simulink model "generate_cartesian_velocity_motion"  (R2025a)
settings: Solver=FixedStepDiscrete  StartTime=0.0  StopTime=inf  FixedStep=0.001  RelTol=1e-3
PreLoadFcn:
  | frs = FrankaRobotSettings();
libraries: simulink x1, franka_simulink x1
settings Model: SimulationMode=external  ExtModeTrigDuration=10000  Creator=vasi_ko  LastModifiedBy=kvasios
settings SolverCC: ConcurrentTasks=on  AlgebraicLoopSolver=TrustRegion
settings DataIOCC: LimitDataPoints=on  SaveFormat=Array  ReturnWorkspaceOutputs=off
settings OptimizationCC: EnhancedBackFolding=on  PassReuseOutputArgsThreshold=0.0  OptimizeBlockOrder=speed  DifferentSizesBufferReuse=on  OptimizationCustomize=off
settings DebuggingCC: SolverPrmCheckMsg=warning  ParameterTunabilityLossMsg=error  UnconnectedInputMsg=warning  UnconnectedOutputMsg=warning  UnconnectedLineMsg=warning  SFUnexpectedBacktrackingDiag=warning  SFNoUnconditionalDefaultTransitionDiag=warning  SFExecutionAtInitializationDiag=none  ArithmeticOperatorsInVariantConditions=warning
settings HardwareCC: ProdBitPerLong=64.0  ProdHWDeviceType=Intel->x86-64 (Linux 64)
settings ModelReferenceCC: EnableRefExpFcnMdlSchedulingChecks=on  PropagateSignalLabelsOutOfModel=off
settings SFSimCC: SimUseLocalCustomCode=off  MATLABDynamicMemAlloc=off  CustomCodeUndefinedFunction=UseInterfaceOnly  SimTargetLang=C++  SimDLTargetLibrary=mkl-dnn
settings RTWCC: HardwareBoard=Generic Linux AMD64 Board  RTWVerbose=off  RTWUseLocalCustomCode=off  BuildConfiguration=Faster Runs  TargetLang=C++  GPUComputeCapability=3.5  DLArmComputeVersion=19.05
settings CodeAppCC: ForceParamTrailComments=on  OperatorAnnotations=on
settings GRTTargetCC: ExtMode=on  ExtModeStaticAlloc=on  ExtModeMexFile=ext_xcp  ExtModeIntrfLevel=Level2 - Open  TargetLangStandard=C++14 (ISO)
settings ConfigComp: CovMetricSettings=dw  CovSaveCumulativeToWorkspaceVar=on  CovSaveSingleToWorkspaceVar=on  CovExternalEMLEnable=off  CovSFcnEnable=off

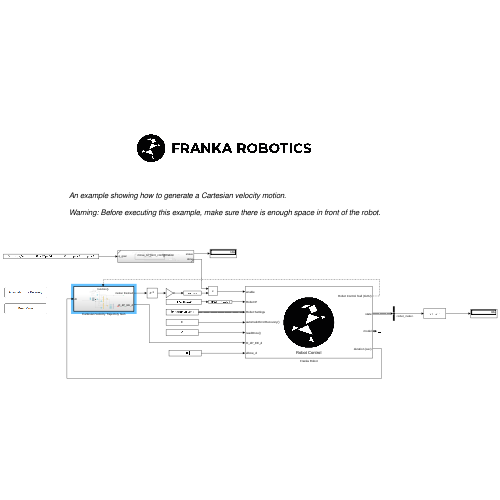
[thumbnail: Simulink's stored preview of the top-level diagram]
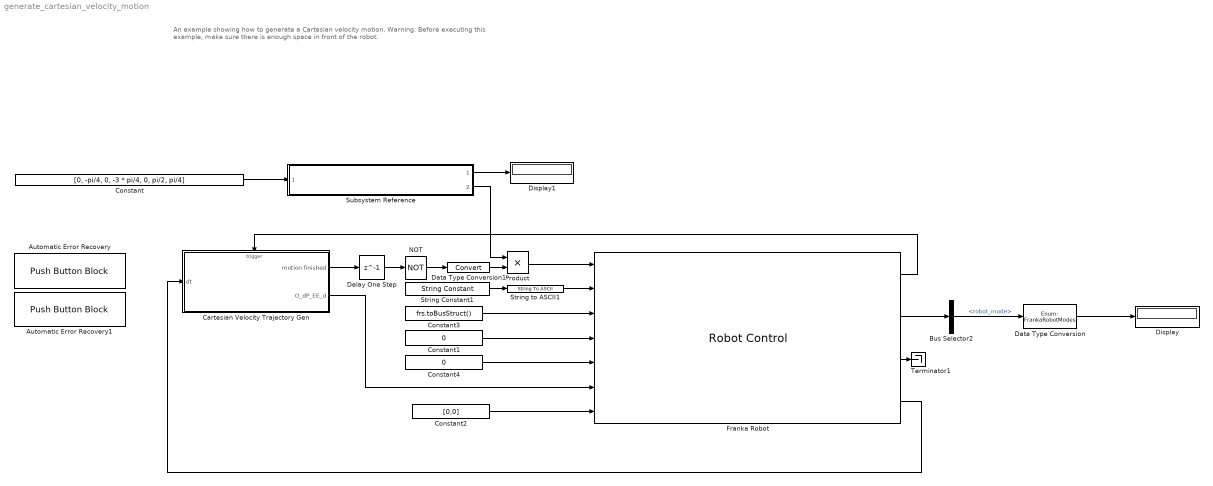
== system generate_cartesian_velocity_motion ==
  note: An example showing how to generate a Cartesian velocity motion.
      |
      | Warning: Before executing this example, make sure there is enough space in front of the robot.
  Automatic Error Recovery : PushButtonBlock  ButtonText=Automatic Error Recovery  IconOnColor=[0.0, 0.39215686274509803, 0.0]  IconOffColor=[0.0, 1.0, 0.0]  OffValue=0.000000
  Automatic Error Recovery1 : PushButtonBlock  ButtonText=Read Once  IconOnColor=[0.0, 0.39215686274509803, 0.0]  IconOffColor=[0.0, 1.0, 0.0]  OffValue=0.000000
  Bus Selector2 : BusSelector  OutputSignals=robot_mode
  Cartesian Velocity Trajectory Gen : Subsystem  TreatAsAtomicUnit=on
      settings: RTWSystemCode=Nonreusable function
  Constant : Constant  Value=[0, -pi/4, 0, -3 * pi/4, 0, pi/2, pi/4]
  Constant1 : Constant  Value=0  OutDataTypeStr=Inherit: Inherit via back propagation
  Constant2 : Constant  Value=[0,0]  OutDataTypeStr=Inherit: Inherit via back propagation
  Constant3 : Constant  Value=frs.toBusStruct()  OutDataTypeStr=Bus: FrankaRobotSettingsBus
  Constant4 : Constant  Value=0  OutDataTypeStr=Inherit: Inherit via back propagation
  Data Type Conversion : DataTypeConversion  OutDataTypeStr=Enum: FrankaRobotModes  SaturateOnIntegerOverflow=off  RndMeth=Floor
  Data Type Conversion1 : DataTypeConversion  SaturateOnIntegerOverflow=off  RndMeth=Floor
  Delay One Step : Delay  DelayLength=1
  Display : Display
  Display1 : Display
  Franka Robot : franka_simulink/Robot Control  control_mode=Cartesian Velocities
      settings: SourceProductName=Franka Robotics Simulink Support Package
  NOT : Logic  Operator=NOT  IconShape=distinctive  AllPortsSameDT=off  OutDataTypeStr=boolean
  Product : Product
  String Constant1 : StringConstant  String="\"172.16.0.2\""
  String to ASCII1 : StringToASCII  OutputVectorSize=16
  Subsystem Reference : Subsystem  ReferencedSubsystem=move_to_joint_configuration
  Terminator1 : Terminator
  wires:
  Subsystem Reference/2 -> Product/1
  Subsystem Reference/1 -> Display1/1
  Constant/1 -> Subsystem Reference/1
  NOT/1 -> Data Type Conversion1/1
  String to ASCII1/1 -> Franka Robot/2
  Bus Selector2/1 -> Data Type Conversion/1  "<robot_mode>"
  String Constant1/1 -> String to ASCII1/1
  Franka Robot/2 -> Bus Selector2/1
  Franka Robot/1 -> Cartesian Velocity Trajectory Gen/Trigger
  Product/1 -> Franka Robot/1
  Constant2/1 -> Franka Robot/7
  Franka Robot/3 -> Terminator1/1
  Data Type Conversion1/1 -> Product/2
  Cartesian Velocity Trajectory Gen/1(motion finished) -> Delay One Step/1
  Data Type Conversion/1 -> Display/1
  Constant1/1 -> Franka Robot/4
  Delay One Step/1 -> NOT/1
  Constant3/1 -> Franka Robot/3
  Cartesian Velocity Trajectory Gen/2(O_dP_EE_d) -> Franka Robot/6
  Franka Robot/4 -> Cartesian Velocity Trajectory Gen/1(dt)
  Constant4/1 -> Franka Robot/5

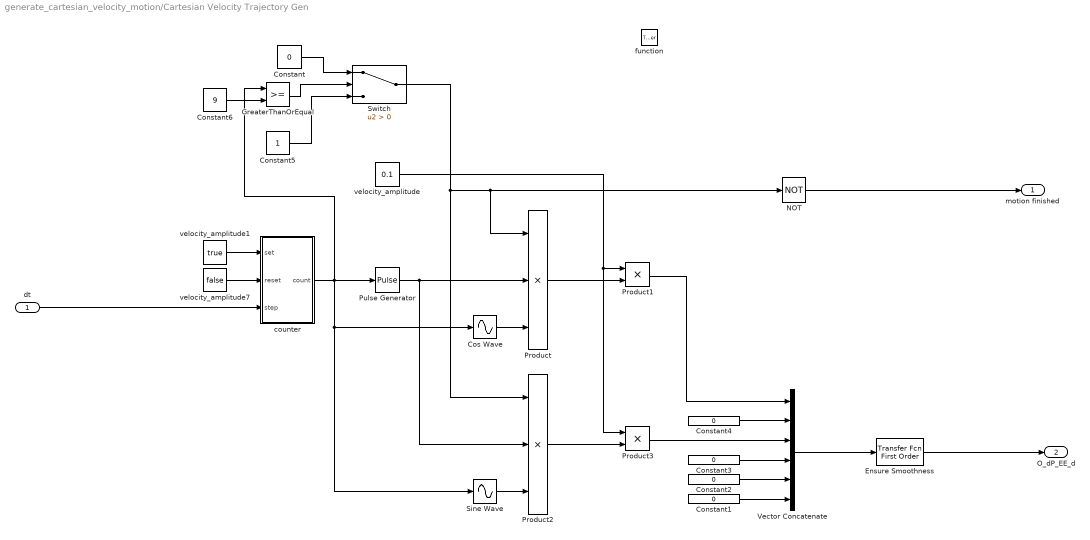
== system generate_cartesian_velocity_motion/Cartesian Velocity Trajectory Gen ==
  dt : Inport
  function : TriggerPort  TriggerType=function-call  VariantControl=(inherit)
  Constant : Constant  Value=0
  Constant{1..4} (4 alike) : Constant  Value=0  VectorParams1D=off
  Constant5 : Constant
  Constant6 : Constant  Value=9
  Cos Wave : Sin  TimeSource=Use external signal  Frequency=pi  Phase=pi+pi/2  SampleTime=0
  Ensure Smoothness : simulink/Discrete/Transfer Fcn First Order  PoleZ=0.99  ICPrevOutput=0.0  DoSatur=off
  GreaterThanOrEqual : RelationalOperator  OutDataTypeStr=boolean  RndMeth=Simplest  InputSameDT=off
  NOT : Logic  Operator=NOT  IconShape=distinctive  AllPortsSameDT=off  OutDataTypeStr=boolean
  Product : Product  Inputs=3
  Product1 : Product
  Product2 : Product  Inputs=3
  Product3 : Product
  Pulse Generator : DiscretePulseGenerator  PulseType=Time based  TimeSource=Use external signal  Period=20  PulseWidth=50  PhaseDelay=1
  Sine Wave : Sin  TimeSource=Use external signal  Frequency=pi  Phase=pi  SampleTime=0
  Switch : Switch  Criteria=u2 > Threshold  SaturateOnIntegerOverflow=off  InputSameDT=off
  Vector Concatenate : Concatenate  NumInputs=6
  counter : Subsystem
  velocity_amplitude : Constant  Value=0.1  VectorParams1D=off
  velocity_amplitude1 : Constant  Value=true  VectorParams1D=off
  velocity_amplitude7 : Constant  Value=false  VectorParams1D=off
  motion finished : Outport  VectorParamsAs1DForOutWhenUnconnected=off
  O_dP_EE_d : Outport  Port=2  VectorParamsAs1DForOutWhenUnconnected=off
  wires:
  Product1/1 -> Vector Concatenate/1
  Product/1 -> Product1/2
  Vector Concatenate/1 -> Ensure Smoothness/1
  Product2/1 -> Product3/2
  Pulse Generator/1 -> Product/2, Product2/2
  Cos Wave/1 -> Product/3
  velocity_amplitude/1 -> Product1/1, Product3/1
  Constant1/1 -> Vector Concatenate/6
  Constant3/1 -> Vector Concatenate/4
  Constant2/1 -> Vector Concatenate/5
  Ensure Smoothness/1 -> O_dP_EE_d/1
  Constant4/1 -> Vector Concatenate/2
  Switch/1 -> Product2/1, Product/1, NOT/1
  Sine Wave/1 -> Product2/3
  NOT/1 -> motion finished/1
  velocity_amplitude7/1 -> counter/2(reset)
  dt/1 -> counter/3(step)
  velocity_amplitude1/1 -> counter/1(set)
  counter/1(count) -> GreaterThanOrEqual/1, Sine Wave/1, Cos Wave/1, Pulse Generator/1
  Product3/1 -> Vector Concatenate/3
  Constant/1 -> Switch/1
  GreaterThanOrEqual/1 -> Switch/2
  Constant5/1 -> Switch/3
  Constant6/1 -> GreaterThanOrEqual/2

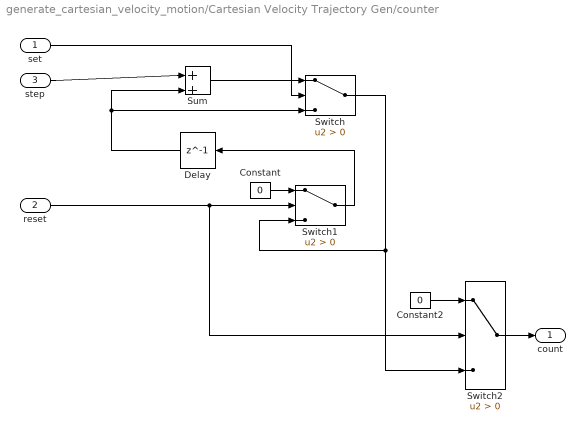
== system generate_cartesian_velocity_motion/Cartesian Velocity Trajectory Gen/counter ==
  set : Inport  OutDataTypeStr=boolean
  reset : Inport  Port=2  OutDataTypeStr=boolean
  step : Inport  Port=3  OutDataTypeStr=double
  Constant : Constant  Value=0  OutDataTypeStr=double
  Constant2 : Constant  Value=0  OutDataTypeStr=double
  Delay : Delay  DelayLength=1  InitialCondition=0
  Sum : Sum  Inputs=|++
  Switch : Switch  Criteria=u2 > Threshold  SaturateOnIntegerOverflow=off  InputSameDT=off
  Switch1 : Switch  Criteria=u2 > Threshold  OutDataTypeStr=double  SaturateOnIntegerOverflow=off  InputSameDT=off
  Switch2 : Switch  Criteria=u2 > Threshold  OutDataTypeStr=double  SaturateOnIntegerOverflow=off  InputSameDT=off
  count : Outport  OutDataTypeStr=double  VectorParamsAs1DForOutWhenUnconnected=off
  wires:
  Switch1/1 -> Delay/1
  Constant/1 -> Switch1/1
  reset/1 -> Switch2/2, Switch1/2
  Delay/1 -> Switch/3, Sum/2
  step/1 -> Sum/1
  Switch/1 -> Switch2/3, Switch1/3
  set/1 -> Switch/2
  Sum/1 -> Switch/1
  Constant2/1 -> Switch2/1
  Switch2/1 -> count/1
